simulink model "edrive"  (R2016b)
settings: Solver=ode1  StartTime=0.0  StopTime=1  FixedStep=ctrlConst.TsSim  MaxStep=1e-6  RelTol=1e-3  EnableMultiTasking=on
PreLoadFcn:
  | %rtwdemo_pmsmfoc_data
StartFcn:
  | %clear executionProfile
StopFcn:
  | %try
  | %  AddExecutionProfileToDataInspector();
  | %end
undefined symbols (not defined in the file or in its folder): canChannel, ctrlConst, ECM, EGM, hm11, hm13, hm5, hm7, Np, pmsm, sensors, sldrtexcb_modeswitch, SpdSetTest, theta0, TrqSetTest, Ts_10ms, Tsw
libraries: powerlib x26, canmsglib x23, simulink x14, canlib x12, powerlib_extras x9
(part 3 of 4)

== system edrive/Motor Control Board/GTM/SVPWMtoDuty/Generate pulse pattern1 ==
  TuHi_On : Inport
  TuHi_Off : Inport  Port=2
  GTM_Hi : MATLAB Function
  Triangle : simulink/Sources/Repeating Sequence  rep_seq_t=[0 1/Fc]  rep_seq_y=[0 1/Fc]
  TuHi : Outport
  wires:
  Triangle/1 -> GTM_Hi/1(Cnt)
  TuHi_On/1 -> GTM_Hi/2(tiOn)
  TuHi_Off/1 -> GTM_Hi/3(tiOff)
  GTM_Hi/1(Port) -> TuHi/1

== system edrive/Motor Control Board/GTM/SVPWMtoDuty/Generate pulse pattern2 ==
  TuHi_On : Inport
  TuHi_Off : Inport  Port=2
  GTM_Hi : MATLAB Function
  Triangle : simulink/Sources/Repeating Sequence  rep_seq_t=[0 1/Fc]  rep_seq_y=[0 1/Fc]
  TuHi : Outport
  wires:
  Triangle/1 -> GTM_Hi/1(Cnt)
  TuHi_On/1 -> GTM_Hi/2(tiOn)
  TuHi_Off/1 -> GTM_Hi/3(tiOff)
  GTM_Hi/1(Port) -> TuHi/1

== system edrive/Motor Control Board/GTM/SVPWMtoDuty/Generate pulse pattern3 ==
  TuLo_Off : Inport
  TuLo_On : Inport  Port=2
  GTM_Lo : MATLAB Function
  Triangle : simulink/Sources/Repeating Sequence  rep_seq_t=[0 1/Fc]  rep_seq_y=[0 1/Fc]
  TuLo : Outport
  wires:
  TuLo_On/1 -> GTM_Lo/3(tiOn)
  Triangle/1 -> GTM_Lo/1(Cnt)
  TuLo_Off/1 -> GTM_Lo/2(tiOff)
  GTM_Lo/1(Port) -> TuLo/1

== system edrive/Motor Control Board/GTM/SVPWMtoDuty/Generate pulse pattern4 ==
  TuLo_Off : Inport
  TuLo_On : Inport  Port=2
  GTM_Lo : MATLAB Function
  Triangle : simulink/Sources/Repeating Sequence  rep_seq_t=[0 1/Fc]  rep_seq_y=[0 1/Fc]
  TuLo : Outport
  wires:
  TuLo_On/1 -> GTM_Lo/3(tiOn)
  Triangle/1 -> GTM_Lo/1(Cnt)
  TuLo_Off/1 -> GTM_Lo/2(tiOff)
  GTM_Lo/1(Port) -> TuLo/1

== system edrive/Motor Control Board/GTM/SVPWMtoDuty/Generate pulse pattern5 ==
  TuLo_Off : Inport
  TuLo_On : Inport  Port=2
  GTM_Lo : MATLAB Function
  Triangle : simulink/Sources/Repeating Sequence  rep_seq_t=[0 1/Fc]  rep_seq_y=[0 1/Fc]
  TuLo : Outport
  wires:
  GTM_Lo/1(Port) -> TuLo/1
  TuLo_Off/1 -> GTM_Lo/2(tiOff)
  Triangle/1 -> GTM_Lo/1(Cnt)
  TuLo_On/1 -> GTM_Lo/3(tiOn)

== system edrive/Motor Control Board/GTM/SVPWMtoDuty/INFO ==
  note: Pattern #2:
      | With this pattern, identified as "Hardware-Determined" by Texas Instruments, there is always one PWM channel staying constant for the entire PWM period.
      |  So the number of switching times for this pattern is less than pattern #1. As a result, switching losses will be reduced with Pattern #2.
  note: Pattern #1:
      | With this pattern, identified as "Software-Determined" by Texas Instruments, each PWM channel switches twice per every PWM period.
  note: --------------------------------------------------------------------------------------------------------------------------------------------------------------------
  note: Reference: Application Report SPRA524
      | Space-Vector PWM with TMS320C24x Using H/W & S/W Determined Switching Patterns
      | Zhenyu Yu, Texas Instruments
  note: The objective of the SV PWM technique is to approximate the reference voltage vector (U*) instantaneously
      | by combination of the switching states corresponding to the basic space vectors.
  note: U7 = 1 1 1
  note: Q1 Q3 Q5
  note: --------------------------------------------------------
  note: Three-Phase VSC Diagram
  note: -
  note: +
  note: --------------------------------------------------------
  note: |
      | |
      | |
  note: ---Vc
  note: |
      | |
      | |
  note: |
      | |
      | |
      | |
      | |
      | |
  note: [Q6]
  note: [Q5]
  note: |
      | |
      | |
  note: ---Vb
  note: |
      | |
      | |
  note: |
      | |
      | |
      | |
      | |
      | |
  note: [Q4]
  note: [Q3]
  note: |
      | |
      | |
  note: ---Va
  note: |
      | |
      | |
  note: |
      | |
      | |
      | |
      | |
      | |
  note: [Q2]
  note: [Q1]
  note: Vdc
  note: [n] = Sector number
  note: [2]
  note: Basic Space Vectors and Switching States
  note: U4 = 0 1 1
  note: U5 = 0 0 1
  note: U6 = 1 0 1
  note: U0 = 0 0 0
  note: U3 = 0 1 0
  note: U2 = 1 1 0
  note: U1 = 1 0 0
  note: [6]
  note: [5]
  note: [4]
  note: [3]
  note: [1]
  note: 3                       2
      |       3                   2
      |         3               2
      |           3           2
      |             3       2
      |               3   2
      | 4 4 4 4 4 4 4 4 0 1 1 1 1 1 1 1 1
      |               5   6
      |             5       6
      |           5           6
      |         5               6
      |       5                   6
      |     5                       6
  note: Two symmetrical switching patterns have been implemented:

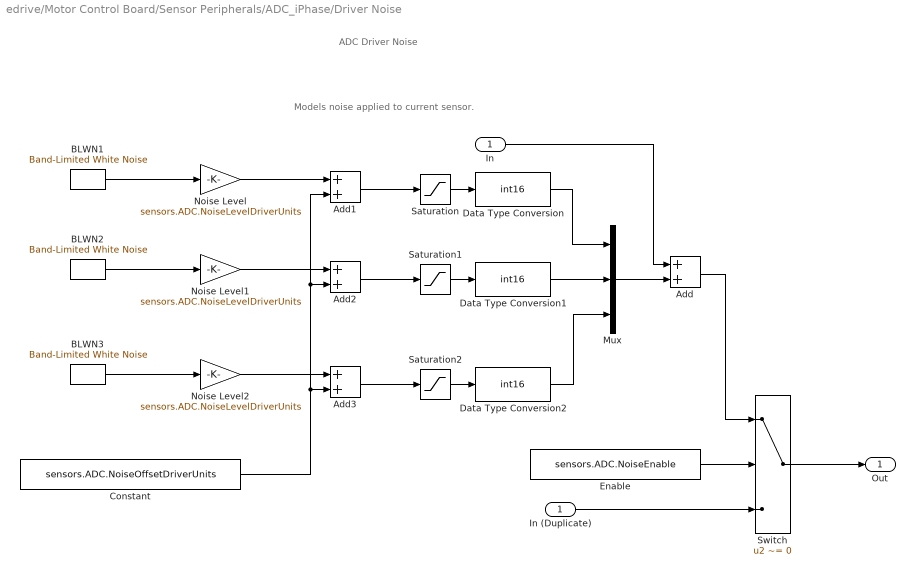
== system edrive/Motor Control Board/Sensor Peripherals/ADC_iPhase/Driver Noise ==
  note: ADC Driver Noise
  note: Models noise applied to current sensor.
  In : Inport
  Add{,1..3} (4 alike) : Sum  RndMeth=Convergent  SaturateOnIntegerOverflow=on
  BLWN1 : simulink/Sources/Band-Limited White Noise  Cov=[(1)^2/10000000]  Ts=ctrlConst.TsSim  seed=[345612]
  BLWN2 : simulink/Sources/Band-Limited White Noise  Cov=[(1)^2/10000000]  Ts=ctrlConst.TsSim  seed=[561234]
  BLWN3 : simulink/Sources/Band-Limited White Noise  Cov=[(1)^2/10000000]  Ts=ctrlConst.TsSim  seed=[123456]
  Constant : Constant  Value=sensors.ADC.NoiseOffsetDriverUnits
  Data Type Conversion : DataTypeConversion  OutDataTypeStr=int16  ConvertRealWorld=Stored Integer (SI)
  Data Type Conversion1 : DataTypeConversion  OutDataTypeStr=int16  ConvertRealWorld=Stored Integer (SI)
  Data Type Conversion2 : DataTypeConversion  OutDataTypeStr=int16  ConvertRealWorld=Stored Integer (SI)
  Enable : Constant  Value=sensors.ADC.NoiseEnable
  In (Duplicate) : InportShadow
  Mux : Mux  Inputs=3
  Noise Level : Gain  Gain=sensors.ADC.NoiseLevelDriverUnits
      settings: AttributesFormatString=------------------------------------\n%<Gain>
  Noise Level1 : Gain  Gain=sensors.ADC.NoiseLevelDriverUnits
      settings: AttributesFormatString=------------------------------------\n%<Gain>
  Noise Level2 : Gain  Gain=sensors.ADC.NoiseLevelDriverUnits
      settings: AttributesFormatString=------------------------------------\n%<Gain>
  Saturation : Saturate  UpperLimit=10  LowerLimit=-10  OutDataTypeStr=double
      settings: AttributesFormatString=----------------------------\nUpper Limit: %<UpperLimit>\nLower Limit: %<LowerLimit>
  Saturation1 : Saturate  UpperLimit=10  LowerLimit=-10  OutDataTypeStr=double
      settings: AttributesFormatString=----------------------------\nUpper Limit: %<UpperLimit>\nLower Limit: %<LowerLimit>
  Saturation2 : Saturate  UpperLimit=10  LowerLimit=-10  OutDataTypeStr=double
      settings: AttributesFormatString=----------------------------\nUpper Limit: %<UpperLimit>\nLower Limit: %<LowerLimit>
  Switch : Switch  Criteria=u2 ~= 0
  Out : Outport
  wires:
  Switch/1 -> Out/1
  BLWN1/1 -> Noise Level/1
  Noise Level/1 -> Add1/1
  Constant/1 -> Add3/2, Add2/2, Add1/2
  Add1/1 -> Saturation/1
  Saturation/1 -> Data Type Conversion/1
  Add/1 -> Switch/1
  In/1 -> Add/1
  In (Duplicate)/1 -> Switch/3
  Enable/1 -> Switch/2
  BLWN2/1 -> Noise Level1/1
  Noise Level1/1 -> Add2/1
  Add2/1 -> Saturation1/1
  Saturation1/1 -> Data Type Conversion1/1
  Add3/1 -> Saturation2/1
  Saturation2/1 -> Data Type Conversion2/1
  Noise Level2/1 -> Add3/1
  BLWN3/1 -> Noise Level2/1
  Mux/1 -> Add/2
  Data Type Conversion1/1 -> Mux/2
  Data Type Conversion2/1 -> Mux/3
  Data Type Conversion/1 -> Mux/1

== system edrive/Motor Control Board/Sensor Peripherals/ADC_uDclink/Driver Noise ==
  note: Models noise applied to current sensor.
  note: ADC Driver Noise
  In : Inport
  Add : Sum  RndMeth=Convergent  SaturateOnIntegerOverflow=on
  Add1 : Sum  RndMeth=Convergent  SaturateOnIntegerOverflow=on
  Constant : Constant  Value=sensors.ADC.NoiseOffsetDriverUnits
  Data Type Conversion : DataTypeConversion  OutDataTypeStr=uint16  RndMeth=Convergent
  Enable : Constant  Value=sensors.ADC.NoiseEnable
  In (Duplicate) : InportShadow
  Noise Level : Gain  Gain=sensors.ADC.NoiseLevelDriverUnits
      settings: AttributesFormatString=------------------------------------\n%<Gain>
  Saturation : Saturate  UpperLimit=sensors.ADC.MaxDriverUnits  LowerLimit=0  OutDataTypeStr=uint16
      settings: AttributesFormatString=----------------------------\nUpper Limit: %<UpperLimit>\nLower Limit: %<LowerLimit>
  Switch : Switch  Criteria=u2 ~= 0
  Uniform Random Number : UniformRandomNumber  Minimum=[0]  Maximum=[1]  SampleTime=ctrlConst.TsSim
  Out : Outport
  wires:
  Enable/1 -> Switch/2
  In (Duplicate)/1 -> Switch/3
  Data Type Conversion/1 -> Add/2
  In/1 -> Add/1
  Add/1 -> Switch/1
  Saturation/1 -> Data Type Conversion/1
  Add1/1 -> Saturation/1
  Constant/1 -> Add1/2
  Noise Level/1 -> Add1/1
  Uniform Random Number/1 -> Noise Level/1
  Switch/1 -> Out/1

== system edrive/Motor Control Board/Sensor Peripherals/BSW_VADC/ADC_Tdbc ==
  u : Inport
  ADC Volts To Driver Units : Constant  Value=sensors.ADC.VoltsToDriverUnits
  Driver Noise : Subsystem
      mask init:
      | if evalin('base','sensors.ADC.NoiseEnable')
      |     enable = 'Enabled';
      | else
      |     enable = 'Disabled';
      | end
      mask Display: fprintf(['ADC Driver Noise\n(' enable ')'])
  Gain : Gain  Gain=16  ParamDataTypeStr=uint16  OutDataTypeStr=uint16
  Product Volts To Driver Units : Product  RndMeth=Zero
  Saturation : Saturate  UpperLimit=sensors.ADC.MaxDriverUnits  LowerLimit=0  OutDataTypeStr=uint16
      settings: AttributesFormatString=----------------------------\nUpper Limit: %<UpperLimit>\nLower Limit: %<LowerLimit>
  ADC : Outport  OutDataTypeStr=uint16
  wires:
  Gain/1 -> ADC/1  "adc_Tdbc"
  Driver Noise/1(Out) -> Gain/1
  Saturation/1 -> Driver Noise/1(In)
  Product Volts To Driver Units/1 -> Saturation/1
  ADC Volts To Driver Units/1 -> Product Volts To Driver Units/2
  u/1 -> Product Volts To Driver Units/1

== system edrive/Motor Control Board/Sensor Peripherals/BSW_VADC/ADC_vdd ==
  u : Inport
  ADC Volts To Driver Units : Constant  Value=sensors.ADC.VoltsToDriverUnits
  Driver Noise : Subsystem
      mask init:
      | if evalin('base','sensors.ADC.NoiseEnable')
      |     enable = 'Enabled';
      | else
      |     enable = 'Disabled';
      | end
      mask Display: fprintf(['ADC Driver Noise\n(' enable ')'])
  Gain : Gain  Gain=16  ParamDataTypeStr=uint16  OutDataTypeStr=uint16
  Product Volts To Driver Units : Product  RndMeth=Zero
  Saturation : Saturate  UpperLimit=sensors.ADC.MaxDriverUnits  LowerLimit=0  OutDataTypeStr=uint16
      settings: AttributesFormatString=----------------------------\nUpper Limit: %<UpperLimit>\nLower Limit: %<LowerLimit>
  ADC : Outport  OutDataTypeStr=uint16
  wires:
  u/1 -> Product Volts To Driver Units/1
  ADC Volts To Driver Units/1 -> Product Volts To Driver Units/2
  Product Volts To Driver Units/1 -> Saturation/1
  Saturation/1 -> Driver Noise/1(In)
  Driver Noise/1(Out) -> Gain/1
  Gain/1 -> ADC/1  "adc_vdd"

== system edrive/Motor Control Board/Sensor Peripherals/BSW_VADC/Tdbc sensor ==
  note: DBC Temperature Sensor
  Bias : Bias  Bias=1
  Constant : Constant  Value=60
  Gain : Gain  Gain=1/200
  NTC : Lookup_n-D  NumberOfTableDimensions=1  BreakpointsForDimension1=[-50:5:150]  BeginIndexSearchUsingPreviousIndexResult=on  Table=[150:-5:-50]  InternalRulePriority=Speed  RndMeth=Simplest  InputSameDT=on
  Vector Concatenate : Concatenate  NumInputs=3
  Vout : Outport
  wires:
  Constant/1 -> Vector Concatenate/3, Vector Concatenate/1, Vector Concatenate/2
  NTC/1 -> Gain/1
  Vector Concatenate/1 -> NTC/1
  Gain/1 -> Bias/1
  Bias/1 -> Vout/1

== system edrive/Motor Control Board/Sensor Peripherals/BSW_VADC/onboard sensor ==
  note: Onboard Voltage Sensor
  Constant : Constant  Value=5
  Constant1 : Constant  Value=14
  Constant2 : Constant  Value=5
  Constant3 : Constant  Value=5
  Gain : Gain  Gain=1/2  SaturateOnIntegerOverflow=on  OutDataTypeStr=Inherit: Same as input  ParamDataTypeStr=Inherit: Same as input
  Gain1 : Gain  Gain=1/5  SaturateOnIntegerOverflow=on  OutDataTypeStr=Inherit: Same as input  ParamDataTypeStr=Inherit: Same as input
  Gain2 : Gain  Gain=1/2  SaturateOnIntegerOverflow=on  OutDataTypeStr=Inherit: Same as input  ParamDataTypeStr=Inherit: Same as input
  Gain3 : Gain  Gain=1/2  SaturateOnIntegerOverflow=on  OutDataTypeStr=Inherit: Same as input  ParamDataTypeStr=Inherit: Same as input
  Vector Concatenate : Concatenate  NumInputs=4
  Vout : Outport
  wires:
  Constant/1 -> Gain/1
  Constant1/1 -> Gain1/1
  Constant2/1 -> Gain2/1
  Constant3/1 -> Gain3/1
  Gain/1 -> Vector Concatenate/1  "vdd5h"
  Gain1/1 -> Vector Concatenate/2  "vdd14"
  Gain2/1 -> Vector Concatenate/3  "vdd5g1"
  Gain3/1 -> Vector Concatenate/4  "vdd5g2"
  Vector Concatenate/1 -> Vout/1

== system edrive/Power Inverter and Motor/Motor_feishi150/PMSM/Continuous ==
  v : Inport
  we : Inport  Port=2
  the : Inport  Port=3
  Constant9 : Constant  Value=120
  Demux : Demux  Outputs=2
  Hall effect sensor : Subsystem
  Mux : Mux
  Mux1 : Mux
  Parameter : Subsystem  TreatAsAtomicUnit=on
  Selector : Selector  InputPortWidth=3  IndexOptions=Index vector (dialog)  Indices=1:2  OutputSizes=1
  "Te " : Fcn  Expr=1.5*Np*(u(3)*u(1)+(u(5)-u(4))*u(1)*u(2))
  Unit Delay : UnitDelay  SampleTime=ctrlConst.TsSim
  abc2qd : Subsystem
  iq,id : Subsystem
  qd2abc : Subsystem
  i : Outport  InitialOutput=0
  m : Outport  Port=2  InitialOutput=0
  Te : Outport  Port=3  InitialOutput=0
  tag scope: Is=global
  wires:
  "Te "/1 -> Te/1
  the/1 -> Hall effect sensor/1(the), abc2qd/2(the), iq,id/2(the)
  we/1 -> Parameter/1(we), iq,id/3(we)
  Mux/1 -> m/1
  abc2qd/2(vq,vd) -> Mux/3, iq,id/1(vq,vd)  "vqd"
  abc2qd/1(s,c) -> qd2abc/1(s,c)
  v/1 -> abc2qd/1(Vab,Vbc)
  iq,id/1(iq,id) -> qd2abc/2(iq,id), Mux1/1, Unit Delay/1, Mux/2  "iqd"
  qd2abc/1(is) -> [Is], Selector/1, Mux/1  "isabc"
  Selector/1 -> i/1
  Hall effect sensor/1(Hall) -> Mux/4  "Hall"
  Parameter/1(Ld) -> iq,id/4(Ld), Mux1/4
  Parameter/2(Lq) -> Mux1/3, iq,id/5(Lq)
  Parameter/3(Rs) -> iq,id/6(Rs)
  Parameter/4(PsiExc) -> iq,id/7(flux), Mux1/2
  Demux/1 -> Parameter/2(Iq)
  Demux/2 -> Parameter/3(Id)
  Constant9/1 -> Parameter/4(Temp)
  Unit Delay/1 -> Demux/1
  Mux1/1 -> "Te "/1

== system edrive/Power Inverter and Motor/Motor_feishi150/PMSM/Continuous w input ==
  In : Inport
  Te : Inport  Port=2
  MotorMode : Inport  Port=3
  Speed : Subsystem
  Switch : Switch  Criteria=u2 > Threshold  Threshold=0.5
  Switch1 : Switch  Criteria=u2 > Threshold  Threshold=0.5
  Switch2 : Switch  Criteria=u2 > Threshold  Threshold=0.5
  Trq : Subsystem
  m : Outport  InitialOutput=0
  we : Outport  Port=2  InitialOutput=0
  the : Outport  Port=3  InitialOutput=0
  wires:
  In/1 -> Trq/1(wm), Speed/1(In)
  Te/1 -> Speed/2(Te), Trq/2(Te)
  MotorMode/1 -> Switch2/2, Switch1/2, Switch/2
  Speed/1(m) -> Switch/1
  Speed/2(we) -> Switch1/1
  Speed/3(the) -> Switch2/1
  Trq/1(m) -> Switch/3
  Trq/2(we) -> Switch1/3
  Trq/3(the) -> Switch2/3
  Switch/1 -> m/1
  Switch1/1 -> we/1
  Switch2/1 -> the/1

== system edrive/Power Inverter and Motor/Motor_feishi150/PMSM/Measurement ==
  m_e : Inport
  m_m : Inport  Port=2
  Bus Creator1 : BusCreator  Inputs=13
  Demux : Demux  Outputs=[1,1,1,1,1,1,1,1,1,1]
  Demux1 : Demux  Outputs=[1,1,1]
  Out1 : Outport
  wires:
  m_m/1 -> Demux1/1
  Bus Creator1/1 -> Out1/1
  m_e/1 -> Demux/1
  Demux/1 -> Bus Creator1/1  "Stator current is_a (A)"
  Demux/2 -> Bus Creator1/2  "Stator current is_b (A)"
  Demux/3 -> Bus Creator1/3  "Stator current is_c (A)"
  Demux/4 -> Bus Creator1/4  "Stator current is_q (A)"
  Demux/5 -> Bus Creator1/5  "Stator current is_d (A)"
  Demux/6 -> Bus Creator1/6  "Stator voltage Vs_q (V)"
  Demux/7 -> Bus Creator1/7  "Stator voltage Vs_d (V)"
  Demux/8 -> Bus Creator1/8  "Hall effect signal h_a"
  Demux/9 -> Bus Creator1/9  "Hall effect signal h_b"
  Demux/10 -> Bus Creator1/10  "Hall effect signal h_c"
  Demux1/1 -> Bus Creator1/11  "Rotor speed wm (rad/s)"
  Demux1/2 -> Bus Creator1/12  "Rotor angle thetam (rad)"
  Demux1/3 -> Bus Creator1/13  "Electromagnetic torque Te (N*m)"

== system edrive/Power Inverter and Motor/Motor_feishi150/PMSM/Powersystem ==
  Controlled Current Source : powerlib/Electrical Sources/Controlled Current Source  Initialize=on  Source_Type=AC  Amplitude=0  Phase=0  Frequency=0  Measurements=None
  Controlled Current Source1 : powerlib/Electrical Sources/Controlled Current Source  Initialize=on  Source_Type=AC  Amplitude=0  Phase=0  Frequency=0  Measurements=None
  Demux : Demux  Outputs=3
  Mux : Mux  Inputs=2
  Terminator3 : Terminator
  Vab_measure : powerlib/Measurements/Voltage Measurement  PhasorSimulation=off  OutputType=Complex  PSBequivalent=0
  Vbc_measure : powerlib/Measurements/Voltage Measurement  PhasorSimulation=off  OutputType=Complex  PSBequivalent=0
  A : PMIOPort  Port=1  Side=Left
  B : PMIOPort  Port=2  Side=Left
  C : PMIOPort  Port=3  Side=Left
  tag scope: UabUbc=global
  wires:
  Vab_measure/1 -> Mux/1
  Vbc_measure/1 -> Mux/2
  Mux/1 -> [UabUbc]
  [Is] -> Demux/1
  Demux/1 -> Controlled Current Source/1
  Demux/3 -> Controlled Current Source1/1
  Demux/2 -> Terminator3/1
  connections:
  B/RConn1 -- Vab_measure/LConn2 -- Vbc_measure/LConn1 -- Controlled Current Source1/RConn1 -- Controlled Current Source/RConn1
  Vbc_measure/LConn2 -- Controlled Current Source1/LConn1 -- C/RConn1
  Controlled Current Source/LConn1 -- Vab_measure/LConn1 -- A/RConn1

== system edrive/System Analysis/Measure/Subsystem4/Subsystem2 ==
  Te : Inport
  wm : Inport  Port=2
  Product1 : Product  RndMeth=Zero
  Transfer Fcn5 : TransferFcn  Denominator=[0.01 1]
  Power1 : Outport
  wires:
  Product1/1 -> Transfer Fcn5/1
  Te/1 -> Product1/1
  wm/1 -> Product1/2
  Transfer Fcn5/1 -> Power1/1

== system edrive/Motor Control Board/Sensor Peripherals/BSW_VADC/ADC_Tdbc/Driver Noise ==
  note: Models noise applied to current sensor.
  note: ADC Driver Noise
  In : Inport
  Add : Sum  RndMeth=Convergent  SaturateOnIntegerOverflow=on
  Add1 : Sum  RndMeth=Convergent  SaturateOnIntegerOverflow=on
  Constant : Constant  Value=sensors.ADC.NoiseOffsetDriverUnits
  Data Type Conversion : DataTypeConversion  OutDataTypeStr=uint16  RndMeth=Convergent
  Enable : Constant  Value=sensors.ADC.NoiseEnable
  In (Duplicate) : InportShadow
  Noise Level : Gain  Gain=sensors.ADC.NoiseLevelDriverUnits
      settings: AttributesFormatString=------------------------------------\n%<Gain>
  Saturation : Saturate  UpperLimit=sensors.ADC.MaxDriverUnits  LowerLimit=0  OutDataTypeStr=uint16
      settings: AttributesFormatString=----------------------------\nUpper Limit: %<UpperLimit>\nLower Limit: %<LowerLimit>
  Switch : Switch  Criteria=u2 ~= 0
  Uniform Random Number : UniformRandomNumber  Minimum=[0 0 0]  Maximum=[1 1 1]  SampleTime=ctrlConst.TsSim
  Out : Outport
  wires:
  Enable/1 -> Switch/2
  In (Duplicate)/1 -> Switch/3
  Data Type Conversion/1 -> Add/2
  In/1 -> Add/1
  Add/1 -> Switch/1
  Saturation/1 -> Data Type Conversion/1
  Add1/1 -> Saturation/1
  Constant/1 -> Add1/2
  Noise Level/1 -> Add1/1
  Uniform Random Number/1 -> Noise Level/1
  Switch/1 -> Out/1

== system edrive/Motor Control Board/Sensor Peripherals/BSW_VADC/ADC_vdd/Driver Noise ==
  note: ADC Driver Noise
  note: Models noise applied to current sensor.
  In : Inport
  Add : Sum  RndMeth=Convergent  SaturateOnIntegerOverflow=on
  Add1 : Sum  RndMeth=Convergent  SaturateOnIntegerOverflow=on
  Constant : Constant  Value=sensors.ADC.NoiseOffsetDriverUnits
  Data Type Conversion : DataTypeConversion  OutDataTypeStr=uint16  RndMeth=Convergent
  Enable : Constant  Value=sensors.ADC.NoiseEnable
  In (Duplicate) : InportShadow
  Noise Level : Gain  Gain=sensors.ADC.NoiseLevelDriverUnits
      settings: AttributesFormatString=------------------------------------\n%<Gain>
  Saturation : Saturate  UpperLimit=sensors.ADC.MaxDriverUnits  LowerLimit=0  OutDataTypeStr=uint16
      settings: AttributesFormatString=----------------------------\nUpper Limit: %<UpperLimit>\nLower Limit: %<LowerLimit>
  Switch : Switch  Criteria=u2 ~= 0
  Uniform Random Number : UniformRandomNumber  Minimum=[0 0 0 0]  Maximum=[1 1 1 1]  SampleTime=ctrlConst.TsSim
  Out : Outport
  wires:
  Switch/1 -> Out/1
  Uniform Random Number/1 -> Noise Level/1
  Noise Level/1 -> Add1/1
  Constant/1 -> Add1/2
  Add1/1 -> Saturation/1
  Saturation/1 -> Data Type Conversion/1
  Add/1 -> Switch/1
  In/1 -> Add/1
  Data Type Conversion/1 -> Add/2
  In (Duplicate)/1 -> Switch/3
  Enable/1 -> Switch/2

== system edrive/Power Inverter and Motor/Motor_feishi150/PMSM/Continuous/Hall effect sensor ==
  the : Inport
  Angle converter : Subsystem
  Constant : Constant  Value=-60
  Constant1 : Constant  Value=120
  Constant2 : Constant  Value=60
  Constant3 : Constant  Value=-120
  Constant4 : Constant  Value=-180
  Constant5 : Constant  Value=0
  Data Type Conversion : DataTypeConversion  OutDataTypeStr=double  SaturateOnIntegerOverflow=on  RndMeth=Zero
  Data Type Conversion1 : DataTypeConversion  OutDataTypeStr=double  SaturateOnIntegerOverflow=on  RndMeth=Zero
  Data Type Conversion2 : DataTypeConversion  OutDataTypeStr=double  SaturateOnIntegerOverflow=on  RndMeth=Zero
  Logical Operator : Logic  AllPortsSameDT=off  OutDataTypeStr=boolean
  Logical Operator1 : Logic  Operator=OR  AllPortsSameDT=off  OutDataTypeStr=boolean
  Logical Operator2 : Logic  AllPortsSameDT=off  OutDataTypeStr=boolean
  Mux : Mux  Inputs=3
  Relational Operator1 : RelationalOperator  Operator=<=  RndMeth=Nearest  InputSameDT=on
  Relational Operator2 : RelationalOperator  RndMeth=Nearest  InputSameDT=on
  Relational Operator3 : RelationalOperator  Operator=<=  RndMeth=Nearest  InputSameDT=on
  Relational Operator4 : RelationalOperator  RndMeth=Nearest  InputSameDT=on
  Relational Operator5 : RelationalOperator  Operator=<=  RndMeth=Nearest  InputSameDT=on
  Relational Operator6 : RelationalOperator  RndMeth=Nearest  InputSameDT=on
  Hall : Outport
  wires:
  the/1 -> Angle converter/1(the)
  Constant3/1 -> Relational Operator3/2
  Constant2/1 -> Relational Operator4/2
  Relational Operator4/1 -> Logical Operator1/1
  Constant1/1 -> Relational Operator1/2
  Constant/1 -> Relational Operator2/2
  Angle converter/1(the_deg) -> Relational Operator4/1, Relational Operator3/1, Relational Operator5/1, Relational Operator6/1, Relational Operator1/1, Relational Operator2/1
  Relational Operator1/1 -> Logical Operator/2
  Relational Operator2/1 -> Logical Operator/1
  Logical Operator/1 -> Data Type Conversion/1
  Logical Operator1/1 -> Data Type Conversion1/1
  Relational Operator3/1 -> Logical Operator1/2
  Constant5/1 -> Relational Operator5/2
  Constant4/1 -> Relational Operator6/2
  Relational Operator6/1 -> Logical Operator2/1
  Logical Operator2/1 -> Data Type Conversion2/1
  Relational Operator5/1 -> Logical Operator2/2
  Data Type Conversion/1 -> Mux/1  "hall 1"
  Data Type Conversion1/1 -> Mux/2  "hall 2"
  Data Type Conversion2/1 -> Mux/3  "hall 3"
  Mux/1 -> Hall/1

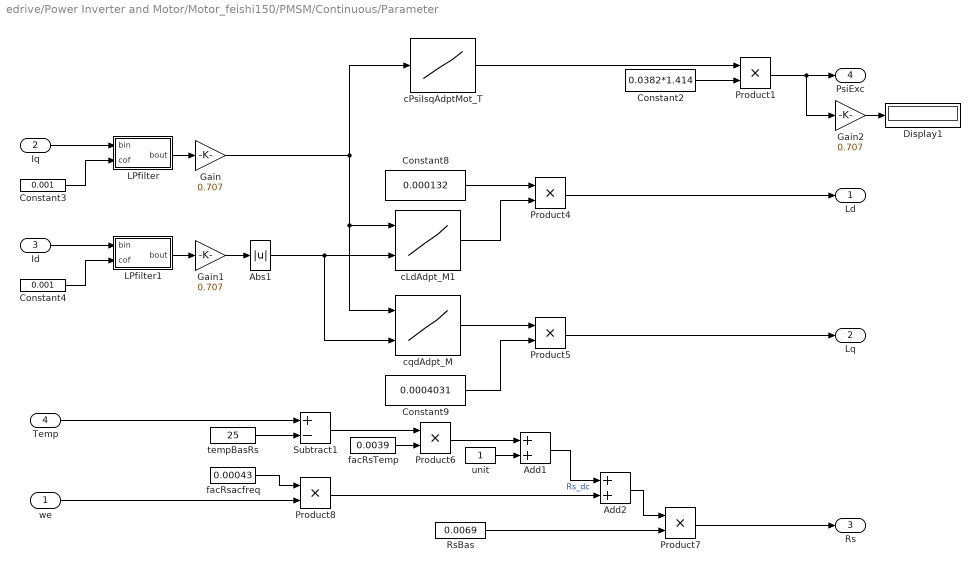
== system edrive/Power Inverter and Motor/Motor_feishi150/PMSM/Continuous/Parameter ==
  we : Inport
  Iq : Inport  Port=2
  Id : Inport  Port=3
  Temp : Inport  Port=4
  Abs1 : Abs
  Add1 : Sum  OutDataTypeStr=Inherit: Same as first input
  Add2 : Sum  OutDataTypeStr=Inherit: Same as first input
  Constant2 : Constant  Value=0.0382*1.414
  Constant3 : Constant  Value=0.001  SampleTime=-1
  Constant4 : Constant  Value=0.001  SampleTime=-1
  Constant8 : Constant  Value=0.000132
  Constant9 : Constant  Value=0.0004031
  Display1 : Display
  Gain : Gain  Gain=0.707
  Gain1 : Gain  Gain=0.707
  Gain2 : Gain  Gain=0.707
  LPfilter : Subsystem  AncestorBlock=PMSM_library/Clarke Transformation  TreatAsAtomicUnit=on
  LPfilter1 : Subsystem  AncestorBlock=PMSM_library/Clarke Transformation  TreatAsAtomicUnit=on
  Product{1,4..8} (6 alike) : Product  RndMeth=Zero
  RsBas : Constant  Value=0.0069  OutDataTypeStr=single  SampleTime=-1
  Subtract1 : Sum  Inputs=+-
  cLdAdpt_M1 : Lookup_n-D  BreakpointsForDimension1=[-550 -500 -450 -400 -350 -300 -250 -200 -150 -100 -50 0 50 100 150 200 250 300 350 400 450 500 550]  BreakpointsForDimension2=|  BeginIndexSearchUsingPreviousIndexResult=on  Table=|  ExtrapMethod=Clip  InternalRulePriority=Speed
      BreakpointsForDimension2=|
      | [0	50	100	150	200	250	300	350	400	450	500	550
      | 
      | ]
      Table=|
      | [0.136363636 0.136363636 0.227272727 0.265151515 0.303030303 0.303030303 0.303030303 0.303030303 0.303030303 0.303030303 0.303030303 0.303030303
      | 0.151515152 0.151515152 0.265151515 0.340909091 0.378787879 0.378787879 0.378787879 0.378787879 0.378787879 0.378787879 0.378787879 0.378787879
      | 0.173280514 0.173280514 0.303030303 0.432780092 0.507575758 0.507575758 0.507575758 0.507575758 0.507575758 0.507575758 0.507575758 0.507575758
      | 0.227791581 0.227791581 0.401515152 0.518027591 0.557321391 0.568181818 0.606060606 0.606060606 0.606060606 0.606060606 0.606060606 0.606060606
      | 0.340909091 0.34540178 0.497391487 0.568719114 0.601368629 0.606060606 0.606060606 0.606060606 0.606060606 0.606060606 0.606060606 0.606060606
      | 0.501270499 0.478030303 0.583333333 0.658420767 0.674673465 0.657778688 0.659090909 0.659090909 0.659090909 0.659090909 0.659090909 0.659090909
      | 0.553787879 0.553787879 0.681818182 0.723317287 0.736910197 0.745065942 0.75 0.75 0.75 0.75 0.75 0.75
      | 0.620975157 0.620975157 0.721939278 0.755593985 0.772421339 0.782517751 0.751006527 0.751006527 0.751006527 0.751006527 0.751006527 0.751006527
      | 0.708809775 0.708809775 0.797506718 0.827072365 0.837333742 0.843490568 0.804115672 0.804115672 0.804115672 0.804115672 0.804115672 0.804115672
      | 0.757575758 0.757575758 0.805818564 0.847685087 0.861836178 0.866709674 0.860496976 0.863636364 0.863636364 0.863636364 0.863636364 0.863636364
      | 0.871212121 0.871212121 0.863636364 0.860088762 0.875660381 0.881386195 0.915384468 0.909090909 0.833333333 0.833333333 0.833333333 0.833333333
      | 0.984848485 0.994718394 0.9856755 0.976632605 0.96080754 0.95312108 0.947503192 0.939393939 0.931818182 0.931818182 0.931818182 0.931818182
      | 0.871212121 0.871212121 0.863636364 0.860088762 0.875660381 0.881386195 0.915384468 0.909090909 0.833333333 0.833333333 0.833333333 0.833333333
      | 0.757575758 0.757575758 0.805818564 0.847685087 0.861836178 0.866709674 0.860496976 0.863636364 0.863636364 0.863636364 0.863636364 0.863636364
      | 0.708809775 0.708809775 0.797506718 0.827072365 0.837333742 0.843490568 0.804115672 0.804115672 0.804115672 0.804115672 0.804115672 0.804115672
      | 0.620975157 0.620975157 0.721939278 0.755593985 0.772421339 0.782517751 0.751006527 0.751006527 0.751006527 0.751006527 0.751006527 0.751006527
      | 0.553787879 0.553787879 0.681818182 0.723317287 0.736910197 0.745065942 0.75 0.75 0.75 0.75 0.75 0.75
      | 0.501270499 0.478030303 0.583333333 0.658420767 0.674673465 0.657778688 0.659090909 0.659090909 0.659090909 0.659090909 0.659090909 0.659090909
      | 0.340909091 0.34540178 0.497391487 0.568719114 0.601368629 0.606060606 0.606060606 0.606060606 0.606060606 0.606060606 0.606060606 0.606060606
      | 0.227791581 0.227791581 0.401515152 0.518027591 0.557321391 0.568181818 0.606060606 0.606060606 0.606060606 0.606060606 0.606060606 0.606060606
      | 0.173280514 0.173280514 0.303030303 0.432780092 0.507575758 0.507575758 0.507575758 0.507575758 0.507575758 0.507575758 0.507575758 0.507575758
      | 0.151515152 0.151515152 0.265151515 0.340909091 0.378787879 0.378787879 0.378787879 0.378787879 0.378787879 0.378787879 0.378787879 0.378787879
      | 0.136363636 0.136363636 0.227272727 0.265151515 0.303030303 0.303030303 0.303030303 0.303030303 0.303030303 0.303030303 0.303030303 0.303030303
      | ]
  cPsiIsqAdptMot_T : Lookup_n-D  NumberOfTableDimensions=1  BreakpointsForDimension1=[-550 -500 -450 -400 -350 -300 -250 -200 -150 -100 -50 0 50 100 150 200 250 300 350 400 450 500 550]  BeginIndexSearchUsingPreviousIndexResult=on  Table=[0.76 0.79 0.818 0.84 0.87 0.9 0.925 0.94 0.958 0.97 0.985 1 0.985 0.97 0.958 0.94 0.925 0.9 0.87 0.84 0.818 0.79 0.76]  ExtrapMethod=Clip  InternalRulePriority=Speed  InputSameDT=on
  cqdAdpt_M : Lookup_n-D  BreakpointsForDimension1=[-550 -500 -450 -400 -350 -300 -250 -200 -150 -100 -50 0 50 100 150 200 250 300 350 400 450 500 550]  BreakpointsForDimension2=|  BeginIndexSearchUsingPreviousIndexResult=on  Table=|  ExtrapMethod=Clip  InternalRulePriority=Speed
      BreakpointsForDimension2=|
      | [0	50	100	150	200	250	300	350	400	450	500	550
      | 
      | ]
      Table=|
      | [0.352269908 0.354750682 0.35971223 0.364673778 0.367154552 0.369635326 0.369635326 0.369635326 0.369635326 0.369635326 0.369635326 0.369635326
      | 0.389481518 0.394443066 0.404366162 0.40932771 0.411808484 0.414289258 0.414289258 0.414289258 0.414289258 0.414289258 0.414289258 0.414289258
      | 0.427291035 0.433739883 0.441577772 0.44653932 0.449020094 0.451500868 0.451500868 0.451500868 0.451500868 0.451500868 0.451500868 0.451500868
      | 0.464909317 0.472164271 0.478432157 0.483712974 0.487019653 0.488712478 0.488712478 0.488712478 0.488712478 0.488712478 0.488712478 0.488712478
      | 0.511019522 0.517054741 0.524782078 0.530253259 0.534032321 0.537811384 0.537811384 0.537811384 0.537811384 0.537811384 0.537811384 0.537811384
      | 0.563945201 0.574325872 0.580001517 0.586368109 0.590168323 0.593228236 0.593228236 0.593228236 0.593228236 0.593228236 0.593228236 0.593228236
      | 0.625998914 0.635889342 0.644595287 0.650340026 0.652531318 0.651761405 0.651761405 0.651761405 0.651761405 0.651761405 0.651761405 0.651761405
      | 0.703286386 0.715649421 0.725791551 0.730751571 0.731269782 0.727346184 0.727666981 0.727666981 0.727666981 0.727666981 0.727666981 0.727666981
      | 0.78965489 0.81008721 0.819661776 0.822326861 0.817095397 0.807915659 0.804395115 0.804395115 0.804395115 0.804395115 0.804395115 0.804395115
      | 0.89280356 0.907165408 0.914124242 0.910718855 0.90287166 0.889102053 0.886782442 0.886782442 0.886782442 0.886782442 0.886782442 0.886782442
      | 0.968314309 0.968314309 0.968314309 0.968314309 0.968314309 0.968314309 0.967501861 0.967501861 0.967501861 0.967501861 0.967501861 0.967501861
      | 0.999999211 0.999999211 0.999999211 0.999999211 0.999999211 0.999999211 0.999999211 0.999999211 0.999999211 0.999999211 0.999999211 0.999999211
      | 0.968314309 0.968314309 0.968314309 0.968314309 0.968314309 0.968314309 0.967501861 0.967501861 0.967501861 0.967501861 0.967501861 0.967501861
      | 0.89280356 0.907165408 0.914124242 0.910718855 0.90287166 0.889102053 0.886782442 0.886782442 0.886782442 0.886782442 0.886782442 0.886782442
      | 0.78965489 0.81008721 0.819661776 0.822326861 0.817095397 0.807915659 0.804395115 0.804395115 0.804395115 0.804395115 0.804395115 0.804395115
      | 0.703286386 0.715649421 0.725791551 0.730751571 0.731269782 0.727346184 0.727666981 0.727666981 0.727666981 0.727666981 0.727666981 0.727666981
      | 0.625998914 0.635889342 0.644595287 0.650340026 0.652531318 0.651761405 0.651761405 0.651761405 0.651761405 0.651761405 0.651761405 0.651761405
      | 0.563945201 0.574325872 0.580001517 0.586368109 0.590168323 0.593228236 0.593228236 0.593228236 0.593228236 0.593228236 0.593228236 0.593228236
      | 0.511019522 0.517054741 0.524782078 0.530253259 0.534032321 0.537811384 0.537811384 0.537811384 0.537811384 0.537811384 0.537811384 0.537811384
      | 0.464909317 0.472164271 0.478432157 0.483712974 0.487019653 0.488712478 0.488712478 0.488712478 0.488712478 0.488712478 0.488712478 0.488712478
      | 0.427291035 0.433739883 0.441577772 0.44653932 0.449020094 0.451500868 0.451500868 0.451500868 0.451500868 0.451500868 0.451500868 0.451500868
      | 0.389481518 0.394443066 0.404366162 0.40932771 0.411808484 0.414289258 0.414289258 0.414289258 0.414289258 0.414289258 0.414289258 0.414289258
      | 0.352269908 0.354750682 0.35971223 0.364673778 0.367154552 0.369635326 0.369635326 0.369635326 0.369635326 0.369635326 0.369635326 0.369635326
      | ]
  facRsTemp : Constant  Value=0.0039  OutDataTypeStr=single  SampleTime=-1
  facRsacfreq : Constant  Value=0.00043  OutDataTypeStr=single  SampleTime=-1
  tempBasRs : Constant  Value=25  OutDataTypeStr=single  SampleTime=-1
  unit : Constant  OutDataTypeStr=single  SampleTime=-1
  Ld : Outport
  Lq : Outport  Port=2
  Rs : Outport  Port=3
  PsiExc : Outport  Port=4
  wires:
  Constant9/1 -> Product5/2
  cqdAdpt_M/1 -> Product5/1
  Constant2/1 -> Product1/2
  cLdAdpt_M1/1 -> Product4/2
  Constant8/1 -> Product4/1
  cPsiIsqAdptMot_T/1 -> Product1/1
  Gain/1 -> cPsiIsqAdptMot_T/1, cqdAdpt_M/1, cLdAdpt_M1/1
  Abs1/1 -> cqdAdpt_M/2, cLdAdpt_M1/2
  Product4/1 -> Ld/1
  Constant3/1 -> LPfilter/2(cof)
  Product7/1 -> Rs/1
  Product5/1 -> Lq/1
  Constant4/1 -> LPfilter1/2(cof)
  LPfilter1/1(bout) -> Gain1/1
  LPfilter/1(bout) -> Gain/1
  Gain1/1 -> Abs1/1
  Iq/1 -> LPfilter/1(bin)
  Id/1 -> LPfilter1/1(bin)
  Gain2/1 -> Display1/1
  Product1/1 -> Gain2/1, PsiExc/1
  RsBas/1 -> Product7/2
  Add1/1 -> Add2/1  "Rs_dc"
  unit/1 -> Add1/2
  Product6/1 -> Add1/1
  facRsTemp/1 -> Product6/2
  Subtract1/1 -> Product6/1
  tempBasRs/1 -> Subtract1/2
  Temp/1 -> Subtract1/1
  we/1 -> Product8/2
  Product8/1 -> Add2/2
  Add2/1 -> Product7/1
  facRsacfreq/1 -> Product8/1

== system edrive/Power Inverter and Motor/Motor_feishi150/PMSM/Continuous/abc2qd ==
  note: This subsystem converts Vab and Vbc to Vd,Vq. The sine and cosine com-
      | puted here are sent to the inverse transformation subsystem dq2abc.
  Vab,Vbc : Inport
  the : Inport  Port=2
  Elementary Math : Trigonometry
  Elementary Math1 : Trigonometry  Operator=cos
  Fcn2 : Fcn  Expr=(u[4]*(2*u[1]+u[2]) + (sqrt(3)*u[2]*u[3])) /3
  Fcn3 : Fcn  Expr=(u[3]*(2*u[1]+u[2]) + (-sqrt(3)*u[2]*u[4])) /3
  Mux1 : Mux  Inputs=[ 2 2 ]
  Mux2 : Mux  Inputs=2
  Mux3 : Mux  Inputs=2
  s,c : Outport  InitialOutput=0
  vq,vd : Outport  Port=2  InitialOutput=0
  wires:
  Mux1/1 -> Fcn2/1, Fcn3/1
  Mux3/1 -> s,c/1, Mux1/2
  Fcn2/1 -> Mux2/1
  Fcn3/1 -> Mux2/2
  Mux2/1 -> vq,vd/1
  Vab,Vbc/1 -> Mux1/1
  the/1 -> Elementary Math/1, Elementary Math1/1
  Elementary Math/1 -> Mux3/1
  Elementary Math1/1 -> Mux3/2

== system edrive/Power Inverter and Motor/Motor_feishi150/PMSM/Continuous/iq,id ==
  vq,vd : Inport
  the : Inport  Port=2
  we : Inport  Port=3
  Ld : Inport  Port=4
  Lq : Inport  Port=5
  Rs : Inport  Port=6
  flux : Inport  Port=7
  Demux : Demux  Outputs=2
  Mux : Mux  Inputs=2
  id : Subsystem
  iq : Subsystem
  iq,id : Outport  InitialOutput=0
  wires:
  id/1(id) -> iq/4(id), Mux/2
  we/1 -> iq/2(we), id/3(we)
  iq/1(iq) -> id/1(iq), Mux/1
  Demux/2 -> id/4(vd)
  Demux/1 -> iq/1(vq)
  vq,vd/1 -> Demux/1
  Mux/1 -> iq,id/1
  Ld/1 -> iq/5(Ld), id/6(Ld)
  Lq/1 -> iq/6(Lq), id/7(Lq)
  Rs/1 -> iq/7(Rs), id/5(Rs)
  flux/1 -> iq/8(flux)
  the/1 -> iq/3(the)
  iq/2(Vd) -> id/2(vd_emf)

== system edrive/Power Inverter and Motor/Motor_feishi150/PMSM/Continuous/qd2abc ==
  s,c : Inport
  iq,id : Inport  Port=2
  Fcn : Fcn  Expr=u[3]*u[2] + u[4]*u[1]
  Fcn1 : Fcn  Expr=(u[2]*(-u[3]-sqrt(3)*u[4]) + u[1]*(sqrt(3)*u[3]-u[4]))*0.5
  Mux : Mux  Inputs=[2,2]
  Mux2 : Mux  Inputs=3
  Sum : Sum  Inputs=--  SaturateOnIntegerOverflow=on  InputSameDT=on  OutDataTypeStr=Inherit: Same as first input
  is : Outport  InitialOutput=0
  wires:
  Mux/1 -> Fcn1/1, Fcn/1
  s,c/1 -> Mux/1
  iq,id/1 -> Mux/2
  Sum/1 -> Mux2/3
  Fcn/1 -> Mux2/1, Sum/2
  Fcn1/1 -> Mux2/2, Sum/1
  Mux2/1 -> is/1

== system edrive/Power Inverter and Motor/Motor_feishi150/PMSM/Continuous w input/Speed ==
  In : Inport
  Te : Inport  Port=2
  Abs : Abs
  Constant : Constant  Value=2*pi
  Fcn2 : Fcn  Expr=(u(1)-theta0)/Np
  FrictionTorque : Lookup_n-D  NumberOfTableDimensions=1  DataSpecification=Lookup table object  LookupTableObject=trqFrcN_T  BreakpointsForDimension1="[0.0\t500.0\t1000.0\t2000.0\t3000.0\t4000.0\t5000.0\t6000.0\t7000.0\t7500.0]"  Table="[2.0\t2.0\t2.25\t2.75\t3.25\t3.75\t4.25\t4.75\t5.25\t5.5]"  ExtrapMethod=Clip  InternalRulePriority=Speed  RndMeth=Simplest
  Gain3 : Gain  Gain=Np  SaturateOnIntegerOverflow=on  OutDataTypeStr=Inherit: Same as input  ParamDataTypeStr=Inherit: Same as input
  Int3 : Integrator
  Math Function : Math  Operator=mod  SaturateOnIntegerOverflow=on
  Mux3 : Mux  Inputs=3
  Subtract : Sum  Inputs=-+
  m : Outport  InitialOutput=0
  we : Outport  Port=2  InitialOutput=0
  the : Outport  Port=3  InitialOutput=0
  wires:
  Gain3/1 -> we/1, Int3/1
  Te/1 -> Subtract/2
  Mux3/1 -> m/1
  In/1 -> Abs/1, Gain3/1, Mux3/1
  Constant/1 -> Math Function/2
  Int3/1 -> Math Function/1, Fcn2/1
  Math Function/1 -> the/1
  Fcn2/1 -> Mux3/2
  Abs/1 -> FrictionTorque/1
  Subtract/1 -> Mux3/3
  FrictionTorque/1 -> Subtract/1

== system edrive/Power Inverter and Motor/Motor_feishi150/PMSM/Continuous w input/Trq ==
  wm : Inport
  Te : Inport  Port=2
  Coulomb & Viscous Friction : simulink/Discontinuities/Coulomb & Viscous Friction  offset=pmsm.Tf  gain=pmsm.F
  Fcn1 : Fcn  Expr=(u(1)-theta0)/Np
  Gain1 : Gain  Gain=Np  SaturateOnIntegerOverflow=on  OutDataTypeStr=Inherit: Same as input  ParamDataTypeStr=Inherit: Same as input
  Gain2 : Gain  Gain=1/pmsm.J  SaturateOnIntegerOverflow=on  OutDataTypeStr=Inherit: Same as input  ParamDataTypeStr=Inherit: Same as input
  Int : Integrator
  Int2 : Integrator  InitialCondition=theta0
  Mux2 : Mux  Inputs=3
  Sum : Sum  Inputs=-+-  SaturateOnIntegerOverflow=on  InputSameDT=on  OutDataTypeStr=Inherit: Same as first input
  m : Outport  InitialOutput=0
  we : Outport  Port=2  InitialOutput=0
  the : Outport  Port=3  InitialOutput=0
  wires:
  wm/1 -> Sum/1
  Int/1 -> Coulomb & Viscous Friction/1, Mux2/1, Gain1/1
  Gain2/1 -> Int/1
  Gain1/1 -> we/1, Int2/1
  Te/1 -> Mux2/3, Sum/2
  Sum/1 -> Gain2/1
  Mux2/1 -> m/1
  Int2/1 -> the/1, Fcn1/1
  Coulomb & Viscous Friction/1 -> Sum/3
  Fcn1/1 -> Mux2/2

== system edrive/Power Inverter and Motor/Motor_feishi150/PMSM/Continuous/Hall effect sensor/Angle converter ==
  note: This subsystem convert 0,infinite angle to -180,180 angle
  the : Inport
  Trigonometric Function : Trigonometry
  Trigonometric Function1 : Trigonometry  Operator=cos
  Trigonometric Function2 : Trigonometry  Operator=atan2
  rad2deg : Gain  Gain=180/pi  SaturateOnIntegerOverflow=on  OutDataTypeStr=Inherit: Same as input  ParamDataTypeStr=Inherit: Same as input
  the_deg : Outport
  wires:
  rad2deg/1 -> the_deg/1
  Trigonometric Function2/1 -> rad2deg/1
  Trigonometric Function1/1 -> Trigonometric Function2/2
  Trigonometric Function/1 -> Trigonometric Function2/1
  the/1 -> Trigonometric Function1/1, Trigonometric Function/1

== system edrive/Power Inverter and Motor/Motor_feishi150/PMSM/Continuous/Parameter/LPfilter ==
  bin : Inport
  cof : Inport  Port=2
  Constant : Constant
  Product1 : Product  RndMeth=Zero
  Product3 : Product  RndMeth=Zero
  Subtract : Sum  Inputs=-+
  Sum1 : Sum  Inputs=|++
  Unit Delay1 : UnitDelay  SampleTime=-1
  bout : Outport
  wires:
  Product3/1 -> Sum1/2
  Unit Delay1/1 -> Product3/1
  Sum1/1 -> Unit Delay1/1, bout/1
  Product1/1 -> Sum1/1
  Subtract/1 -> Product3/2
  bin/1 -> Product1/1
  Constant/1 -> Subtract/2
  cof/1 -> Subtract/1, Product1/2

== system edrive/Power Inverter and Motor/Motor_feishi150/PMSM/Continuous/Parameter/LPfilter1 ==
  bin : Inport
  cof : Inport  Port=2
  Constant : Constant
  Product1 : Product  RndMeth=Zero
  Product3 : Product  RndMeth=Zero
  Subtract : Sum  Inputs=-+
  Sum1 : Sum  Inputs=|++
  Unit Delay1 : UnitDelay  SampleTime=-1
  bout : Outport
  wires:
  Product3/1 -> Sum1/2
  Unit Delay1/1 -> Product3/1
  Sum1/1 -> Unit Delay1/1, bout/1
  Product1/1 -> Sum1/1
  Subtract/1 -> Product3/2
  bin/1 -> Product1/1
  Constant/1 -> Subtract/2
  cof/1 -> Subtract/1, Product1/2

== system edrive/Power Inverter and Motor/Motor_feishi150/PMSM/Continuous/iq,id/id ==
  iq : Inport
  vd_emf : Inport  Port=2
  we : Inport  Port=3
  vd : Inport  Port=4
  Rs : Inport  Port=5
  Ld : Inport  Port=6
  Lq : Inport  Port=7
  Product : Product  SaturateOnIntegerOverflow=on  InputSameDT=on  OutDataTypeStr=Inherit: Same as first input
  Product1 : Product  Inputs=*/  SaturateOnIntegerOverflow=on  InputSameDT=on  OutDataTypeStr=Inherit: Same as first input
  Product2 : Product  Inputs=**/  SaturateOnIntegerOverflow=on  InputSameDT=on  OutDataTypeStr=Inherit: Same as first input
  Product3 : Product  Inputs=**/  SaturateOnIntegerOverflow=on  InputSameDT=on  OutDataTypeStr=Inherit: Same as first input
  Product4 : Product  Inputs=*/  SaturateOnIntegerOverflow=on  InputSameDT=on  OutDataTypeStr=Inherit: Same as first input
  Sum : Sum  Inputs=--++  SaturateOnIntegerOverflow=on  InputSameDT=on  OutDataTypeStr=Inherit: Same as first input
  "id " : Integrator
  id : Outport  InitialOutput=0
  wires:
  iq/1 -> Product/2
  we/1 -> Product/1
  vd/1 -> Product1/1
  "id "/1 -> Product2/1, id/1
  Product/1 -> Product3/1
  Sum/1 -> "id "/1
  Product3/1 -> Sum/4
  Product2/1 -> Sum/1
  Product1/1 -> Sum/3
  Rs/1 -> Product2/2
  Ld/1 -> Product4/2, Product3/3, Product1/2, Product2/3
  Lq/1 -> Product3/2
  vd_emf/1 -> Product4/1
  Product4/1 -> Sum/2

== system edrive/Power Inverter and Motor/Motor_feishi150/PMSM/Continuous/iq,id/iq ==
  vq : Inport
  we : Inport  Port=2
  the : Inport  Port=3
  id : Inport  Port=4
  Ld : Inport  Port=5
  Lq : Inport  Port=6
  Rs : Inport  Port=7
  flux : Inport  Port=8
  Constant2 : Constant
  Product1 : Product  SaturateOnIntegerOverflow=on  InputSameDT=on  OutDataTypeStr=Inherit: Same as first input
  Product2 : Product  Inputs=**/  SaturateOnIntegerOverflow=on  InputSameDT=on  OutDataTypeStr=Inherit: Same as first input
  Product3 : Product  Inputs=**/  SaturateOnIntegerOverflow=on  InputSameDT=on  OutDataTypeStr=Inherit: Same as first input
  Product4 : Product  Inputs=*/  SaturateOnIntegerOverflow=on  InputSameDT=on  OutDataTypeStr=Inherit: Same as first input
  Product5 : Product  Inputs=**/  SaturateOnIntegerOverflow=on  InputSameDT=on  OutDataTypeStr=Inherit: Same as first input
  Subsystem : Subsystem
  Sum1 : Sum  Inputs=---+  SaturateOnIntegerOverflow=on  InputSameDT=on  OutDataTypeStr=Inherit: Same as first input
  "iq " : Integrator
  iq : Outport  InitialOutput=0
  Vd : Outport  Port=2  InitialOutput=0
  wires:
  "iq "/1 -> Product3/1, iq/1
  we/1 -> Subsystem/1(we), Product1/2
  vq/1 -> Product4/1
  id/1 -> Product1/1
  Product4/1 -> Sum1/4
  Product1/1 -> Product2/1
  Sum1/1 -> "iq "/1
  Product5/1 -> Sum1/3
  Product2/1 -> Sum1/2
  Product3/1 -> Sum1/1
  Ld/1 -> Product2/2
  Lq/1 -> Product3/3, Product4/2, Product5/3, Product2/3
  Rs/1 -> Product3/2
  flux/1 -> Subsystem/3(flux)
  the/1 -> Subsystem/2(the)
  Subsystem/2(Vd) -> Vd/1
  Constant2/1 -> Product5/1
  Subsystem/1(Vq) -> Product5/2
